simulink model "SprottD_XSG"  (R2020a)
settings: Solver=VariableStepAuto  StartTime=0.0  StopTime=500  RelTol=1e-3
libraries: xbsIndex_r4 x24
settings Model: Creator=RaviM  LastModifiedBy=RaviM

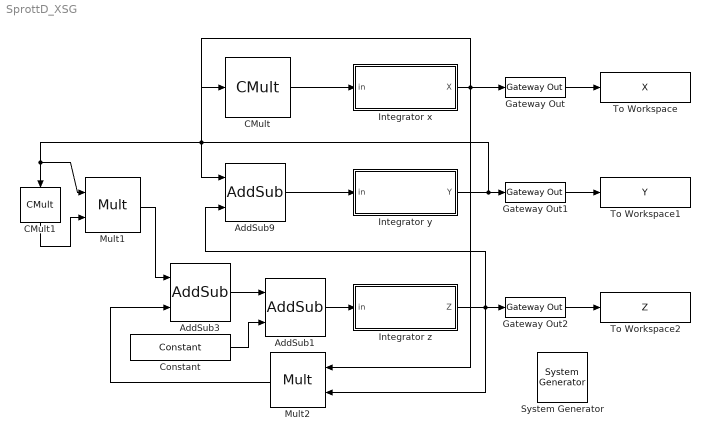
== system SprottD_XSG ==
  " System Generator" : xbsIndex_r4/ System Generator  Tag=genX  xilinxfamily=artix7  part=xc7a35t  speed=-1  package=cpg236  synthesis_tool=Vivado  clock_wrapper=Clock Enables  directory=./netlist/sprottD  proj_type=Vivado  Synth_file=Vivado Synthesis Defaults  Impl_file=Vivado Implementation Defaults  testbench=on  simulink_period=1/100  sysclk_period=10  dcm_input_clock_period=10  incr_netlist=off  trim_vbits=Everywhere in SubSystem  dbl_ovrd=According to Block Masks  core_generation=According to Block Masks  run_coregen=off  deprecated_control=off  eval_field=0  block_type=sysgen
  AddSub1 : xbsIndex_r4/AddSub  mode=Subtraction  use_carryin=off  use_carryout=off  en=off  latency=0  precision=User Defined  arith_type="Signed  (2's comp)"  n_bits=32  bin_pt=24  quantization=Truncate  overflow=Wrap  use_behavioral_HDL=off  hw_selection=DSP48  pipelined=off  dbl_ovrd=off  block_type=addsub
  AddSub3 : xbsIndex_r4/AddSub  mode=Addition  use_carryin=off  use_carryout=off  en=off  latency=0  precision=User Defined  arith_type="Signed  (2's comp)"  n_bits=32  bin_pt=24  quantization=Truncate  overflow=Wrap  use_behavioral_HDL=off  hw_selection=DSP48  pipelined=off  dbl_ovrd=off  block_type=addsub
  AddSub9 : xbsIndex_r4/AddSub  mode=Addition  use_carryin=off  use_carryout=off  en=off  latency=0  precision=User Defined  arith_type="Signed  (2's comp)"  n_bits=32  bin_pt=24  quantization=Truncate  overflow=Wrap  use_behavioral_HDL=off  hw_selection=DSP48  pipelined=off  dbl_ovrd=off  block_type=addsub
  CMult : xbsIndex_r4/CMult  const=-1  gui_display_data_type=Fixed-point  const_n_bits=32  const_bin_pt=24  float_type=Single  exp_bits=8  fraction_bits=24  en=off  latency=0  precision=User Defined  arith_type="Signed  (2's comp)"  n_bits=32  bin_pt=24  quantization=Truncate  overflow=Wrap  use_behavioral_HDL=off  mem_type=Distributed RAM  pipeline=off  dbl_ovrd=off  block_type=cmult
  CMult1 : xbsIndex_r4/CMult  const=2  gui_display_data_type=Fixed-point  const_n_bits=32  const_bin_pt=24  float_type=Single  exp_bits=8  fraction_bits=24  en=off  latency=0  precision=User Defined  arith_type="Signed  (2's comp)"  n_bits=32  bin_pt=24  quantization=Truncate  overflow=Wrap  use_behavioral_HDL=off  mem_type=Distributed RAM  pipeline=off  dbl_ovrd=off  block_type=cmult
  Constant : xbsIndex_r4/Constant  const=0.2  gui_display_data_type=Fixed-point  arith_type=Signed (2's comp)  n_bits=32  bin_pt=24  preci_type=Single  exp_width=8  frac_width=24  explicit_period=on  period=1  equ=P=C  opselect=C  inp2=PCIN>>17  opr=+  inp1=P  carry=CIN  dbl_ovrd=off  block_type=constant
  Gateway Out : xbsIndex_r4/Gateway Out  inherit_from_input=off  hdl_port=on  rows=1  columns=1  UseAsDAC=off  DACChannel='1'  interface=None  automatic_assignment=on  address_offset=hex2dec('00')  intf_name=''  intf_description=''  timing_constraint=None  locs_specified=off  LOCs={}  io_standard={}  block_type=gatewayout
  Gateway Out1 : xbsIndex_r4/Gateway Out  inherit_from_input=off  hdl_port=on  rows=1  columns=1  UseAsDAC=off  DACChannel='1'  interface=None  automatic_assignment=on  address_offset=hex2dec('00')  intf_name=''  intf_description=''  timing_constraint=None  locs_specified=off  LOCs={}  io_standard={}  block_type=gatewayout
  Gateway Out2 : xbsIndex_r4/Gateway Out  inherit_from_input=off  hdl_port=on  rows=1  columns=1  UseAsDAC=off  DACChannel='1'  interface=None  automatic_assignment=on  address_offset=hex2dec('00')  intf_name=''  intf_description=''  timing_constraint=None  locs_specified=off  LOCs={}  io_standard={}  block_type=gatewayout
  Integrator x : Subsystem
  Integrator y : Subsystem
  Integrator z : Subsystem
  Mult1 : xbsIndex_r4/Mult  precision=User Defined  arith_type="Signed  (2's comp)"  n_bits=32  bin_pt=24  quantization=Truncate  overflow=Wrap  en=off  latency=0  use_behavioral_HDL=off  opt=Speed  use_embedded=on  optimum_pipeline=off  pipeline=on  dbl_ovrd=off  use_rpm=on  placement_style=Triangular  block_type=mult
  Mult2 : xbsIndex_r4/Mult  precision=User Defined  arith_type="Signed  (2's comp)"  n_bits=32  bin_pt=24  quantization=Truncate  overflow=Wrap  en=off  latency=0  use_behavioral_HDL=off  opt=Speed  use_embedded=on  optimum_pipeline=off  pipeline=on  dbl_ovrd=off  use_rpm=on  placement_style=Triangular  block_type=mult
  To Workspace : ToWorkspace  VariableName=X  SaveFormat=Timeseries  SampleTime=-1
  To Workspace1 : ToWorkspace  VariableName=Y  SaveFormat=Timeseries  SampleTime=-1
  To Workspace2 : ToWorkspace  VariableName=Z  SaveFormat=Timeseries  SampleTime=-1
  wires:
  CMult/1 -> Integrator x/1(in)
  Integrator x/1(X) -> AddSub9/1, Gateway Out/1, Mult2/1
  Integrator y/1(Y) -> Gateway Out1/1, CMult1/1, Mult1/1, CMult/1
  Integrator z/1(Z) -> AddSub9/2, Mult2/2, Gateway Out2/1
  AddSub9/1 -> Integrator y/1(in)
  CMult1/1 -> Mult1/2
  Mult1/1 -> AddSub3/1
  Mult2/1 -> AddSub3/2
  AddSub3/1 -> AddSub1/1
  Constant/1 -> AddSub1/2
  AddSub1/1 -> Integrator z/1(in)
  Gateway Out2/1 -> To Workspace2/1
  Gateway Out1/1 -> To Workspace1/1
  Gateway Out/1 -> To Workspace/1

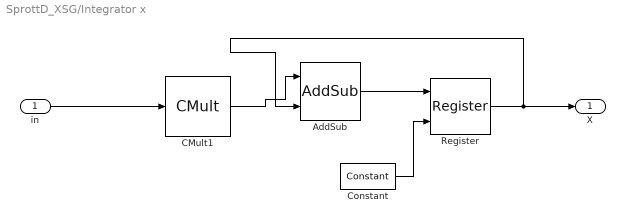
== system SprottD_XSG/Integrator x ==
  in : Inport
  AddSub : xbsIndex_r4/AddSub  mode=Addition  use_carryin=off  use_carryout=off  en=off  latency=0  precision=User Defined  arith_type="Signed  (2's comp)"  n_bits=32  bin_pt=24  quantization=Truncate  overflow=Wrap  use_behavioral_HDL=off  hw_selection=DSP48  pipelined=off  dbl_ovrd=off  block_type=addsub
  CMult1 : xbsIndex_r4/CMult  const=0.01  gui_display_data_type=Fixed-point  const_n_bits=32  const_bin_pt=24  float_type=Single  exp_bits=8  fraction_bits=24  en=off  latency=0  precision=User Defined  arith_type="Signed  (2's comp)"  n_bits=32  bin_pt=24  quantization=Truncate  overflow=Wrap  use_behavioral_HDL=off  mem_type=Distributed RAM  pipeline=off  dbl_ovrd=off  block_type=cmult
  Constant : xbsIndex_r4/Constant  const=0  gui_display_data_type=Boolean  arith_type=Boolean  n_bits=16  bin_pt=14  preci_type=Single  exp_width=8  frac_width=24  explicit_period=on  period=0.01  equ=P=C  opselect=C  inp2=PCIN>>17  opr=+  inp1=P  carry=CIN  dbl_ovrd=off  block_type=constant
  Register : xbsIndex_r4/Register  init=0.1  rst=on  en=off  dbl_ovrd=off  block_type=register
      settings: block_version=11.1
  X : Outport  SampleTime=0.01
  wires:
  CMult1/1 -> AddSub/1
  AddSub/1 -> Register/1
  Register/1 -> X/1, AddSub/2
  in/1 -> CMult1/1
  Constant/1 -> Register/2

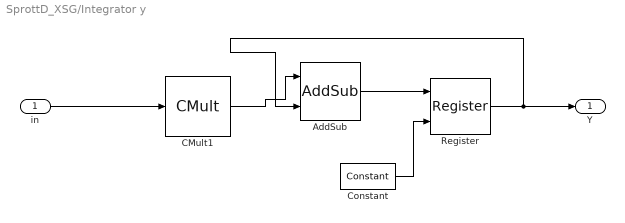
== system SprottD_XSG/Integrator y ==
  in : Inport
  AddSub : xbsIndex_r4/AddSub  mode=Addition  use_carryin=off  use_carryout=off  en=off  latency=0  precision=User Defined  arith_type="Signed  (2's comp)"  n_bits=32  bin_pt=24  quantization=Truncate  overflow=Wrap  use_behavioral_HDL=off  hw_selection=DSP48  pipelined=off  dbl_ovrd=off  block_type=addsub
  CMult1 : xbsIndex_r4/CMult  const=0.01  gui_display_data_type=Fixed-point  const_n_bits=32  const_bin_pt=24  float_type=Single  exp_bits=8  fraction_bits=24  en=off  latency=0  precision=User Defined  arith_type="Signed  (2's comp)"  n_bits=32  bin_pt=24  quantization=Truncate  overflow=Wrap  use_behavioral_HDL=off  mem_type=Distributed RAM  pipeline=off  dbl_ovrd=off  block_type=cmult
  Constant : xbsIndex_r4/Constant  const=0  gui_display_data_type=Boolean  arith_type=Boolean  n_bits=16  bin_pt=14  preci_type=Single  exp_width=8  frac_width=24  explicit_period=on  period=0.01  equ=P=C  opselect=C  inp2=PCIN>>17  opr=+  inp1=P  carry=CIN  dbl_ovrd=off  block_type=constant
  Register : xbsIndex_r4/Register  init=0.7  rst=on  en=off  dbl_ovrd=off  block_type=register
  Y : Outport
  wires:
  in/1 -> CMult1/1
  AddSub/1 -> Register/1
  Constant/1 -> Register/2
  CMult1/1 -> AddSub/1
  Register/1 -> Y/1, AddSub/2

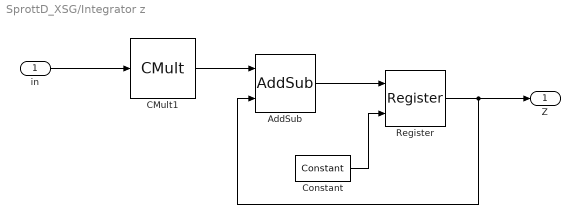
== system SprottD_XSG/Integrator z ==
  in : Inport
  AddSub : xbsIndex_r4/AddSub  mode=Addition  use_carryin=off  use_carryout=off  en=off  latency=0  precision=User Defined  arith_type="Signed  (2's comp)"  n_bits=32  bin_pt=24  quantization=Truncate  overflow=Wrap  use_behavioral_HDL=off  hw_selection=DSP48  pipelined=off  dbl_ovrd=off  block_type=addsub
  CMult1 : xbsIndex_r4/CMult  const=0.01  gui_display_data_type=Fixed-point  const_n_bits=32  const_bin_pt=24  float_type=Single  exp_bits=8  fraction_bits=24  en=off  latency=0  precision=User Defined  arith_type="Signed  (2's comp)"  n_bits=32  bin_pt=24  quantization=Truncate  overflow=Wrap  use_behavioral_HDL=off  mem_type=Distributed RAM  pipeline=off  dbl_ovrd=off  block_type=cmult
  Constant : xbsIndex_r4/Constant  const=0  gui_display_data_type=Boolean  arith_type=Boolean  n_bits=16  bin_pt=14  preci_type=Single  exp_width=8  frac_width=24  explicit_period=on  period=0.01  equ=P=C  opselect=C  inp2=PCIN>>17  opr=+  inp1=P  carry=CIN  dbl_ovrd=off  block_type=constant
  Register : xbsIndex_r4/Register  init=0.4  rst=on  en=off  dbl_ovrd=off  block_type=register
  Z : Outport
  wires:
  in/1 -> CMult1/1
  AddSub/1 -> Register/1
  Constant/1 -> Register/2
  CMult1/1 -> AddSub/1
  Register/1 -> Z/1, AddSub/2
